simulink model "Reactive_System_Wiper"  (R2024b)
settings: Solver=FixedStepDiscrete  StartTime=0.0  StopTime=10.0  RelTol=1e-3
undefined symbols (not defined in the file or in its folder): APP_Modes
settings Model: Creator=Ahmad  LastModifiedBy=Ahmad
settings OptimizationCC: DefaultParameterBehavior=Inlined  UseDivisionForNetSlopeComputation=on  GainParamInheritBuiltInType=on  UseFloatMulNetSlope=on  InlineInvariantSignals=on  PassReuseOutputArgsAs=Individual arguments  ZeroExternalMemoryAtStartup=off  ZeroInternalMemoryAtStartup=off  NoFixptDivByZeroProtection=on  EfficientFloat2IntCast=on  LifeSpan=1  OptimizeBlockOrder=speed  DifferentSizesBufferReuse=on  EfficientTunableParamExpr=on
settings DebuggingCC: ParameterTunabilityLossMsg=error
settings HardwareCC: ProdBitPerInt=16  ProdBitPerPointer=16  ProdBitPerSizeT=16  ProdBitPerPtrDiffT=16  ProdLargestAtomicFloat=None  ProdWordSize=16  ProdLongLongMode=on  ProdHWDeviceType=STMicroelectronics->ST10/Super10
settings SFSimCC: MATLABDynamicMemAlloc=off
settings RTWCC: Description=Embedded Coder  SystemTargetFile=ert.tlc  TemplateMakefile=ert_default_tmf
settings CodeAppCC: ForceParamTrailComments=on  IgnoreCustomStorageClasses=off  OperatorAnnotations=on  SimulinkDataObjDesc=on  SFDataObjDesc=on  CustomSymbolStrGlobalVar=rt$N$M  CustomSymbolStrType=$N$M  CustomSymbolStrFcn=$N$M$F  CustomSymbolStrMacro=$N$M  InsertBlockDesc=on
settings ERTTargetCC: TargetLangStandard=C99 (ISO)  GenerateSampleERTMain=on  IncludeMdlTerminateFcn=off  CombineSignalStateStructs=on  SuppressErrorStatus=on  SupportAbsoluteTime=off  SupportComplex=off  ERTCustomFileTemplate=example_file_process.tlc  ERTFilePackagingFormat=CompactWithDataFile

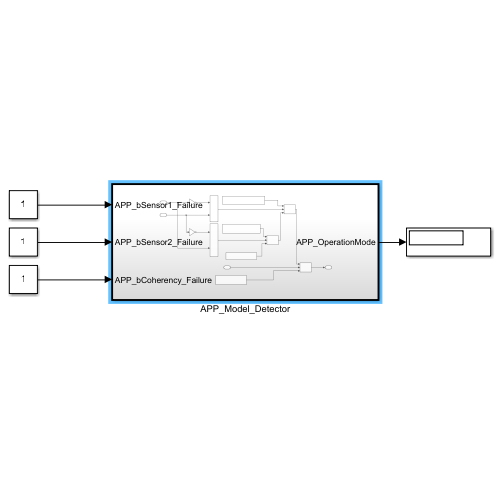
[thumbnail: Simulink's stored preview of the top-level diagram]
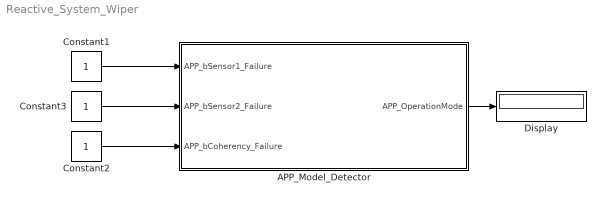
== system Reactive_System_Wiper ==
  APP_Model_Detector : Subsystem  TreatAsAtomicUnit=on
  Constant1 : Constant  OutDataTypeStr=single
  Constant2 : Constant  OutDataTypeStr=single
  Constant3 : Constant  OutDataTypeStr=single
  Display : Display
  wires:
  Constant1/1 -> APP_Model_Detector/1(APP_bSensor1_Failure)
  Constant2/1 -> APP_Model_Detector/3(APP_bCoherency_Failure)
  Constant3/1 -> APP_Model_Detector/2(APP_bSensor2_Failure)
  APP_Model_Detector/1(APP_OperationMode) -> Display/1

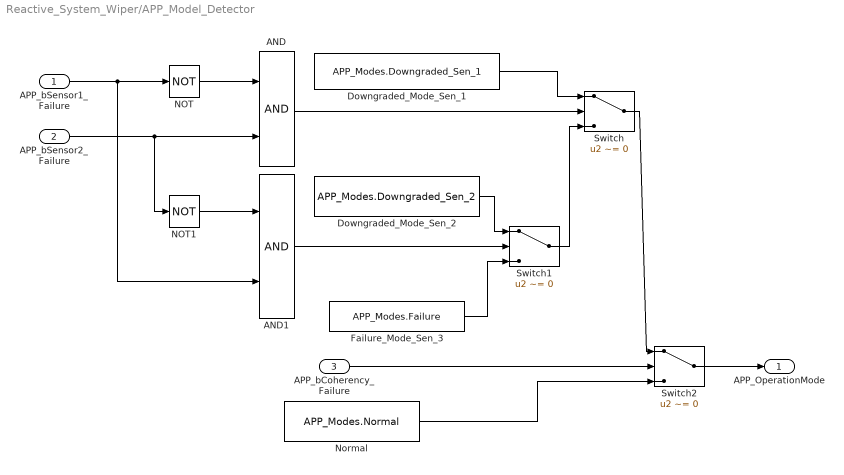
== system Reactive_System_Wiper/APP_Model_Detector ==
  APP_bSensor1_Failure : Inport
  APP_bSensor2_Failure : Inport  Port=2
  APP_bCoherency_Failure : Inport  Port=3
  AND : Logic  AllPortsSameDT=off  OutDataTypeStr=boolean
  AND1 : Logic  AllPortsSameDT=off  OutDataTypeStr=boolean
  Downgraded_Mode_Sen_1 : Constant  Value=APP_Modes.Downgraded_Sen_1
  Downgraded_Mode_Sen_2 : Constant  Value=APP_Modes.Downgraded_Sen_2  LockScale=on
  Failure_Mode_Sen_3 : Constant  Value=APP_Modes.Failure
  NOT : Logic  Operator=NOT  IconShape=distinctive  AllPortsSameDT=off  OutDataTypeStr=boolean
  NOT1 : Logic  Operator=NOT  IconShape=distinctive  AllPortsSameDT=off  OutDataTypeStr=boolean
  Normal : Constant  Value=APP_Modes.Normal
  Switch : Switch  Criteria=u2 ~= 0  SaturateOnIntegerOverflow=off  InputSameDT=off
  Switch1 : Switch  Criteria=u2 ~= 0  SaturateOnIntegerOverflow=off  InputSameDT=off
  Switch2 : Switch  Criteria=u2 ~= 0  SaturateOnIntegerOverflow=off  InputSameDT=off
  APP_OperationMode : Outport
  wires:
  NOT/1 -> AND/1
  APP_bSensor1_Failure/1 -> AND1/2, NOT/1
  APP_bSensor2_Failure/1 -> NOT1/1, AND/2
  NOT1/1 -> AND1/1
  Downgraded_Mode_Sen_1/1 -> Switch/1
  AND/1 -> Switch/2
  AND1/1 -> Switch1/2
  Downgraded_Mode_Sen_2/1 -> Switch1/1
  Failure_Mode_Sen_3/1 -> Switch1/3
  Switch1/1 -> Switch/3
  APP_bCoherency_Failure/1 -> Switch2/2
  Normal/1 -> Switch2/3
  Switch/1 -> Switch2/1
  Switch2/1 -> APP_OperationMode/1
